simulink model "pid_bdc_z_sim"  (R2025b)
settings: Solver=ode45  StartTime=0.0  StopTime=0.5  MaxStep=0.001  RelTol=1e-3
values from neighbouring files (symbols this model uses):
  A = [-Ra/La, -Kb/La, 0 ; Kb/Je, -Be/Je, 0 ; 0, 1, 0]    [pid_bdc_z.m]
  B = [1/La ; 0 ; 0]    [pid_bdc_z.m]
  C = [0, 0, 1]    [pid_bdc_z.m]
  D = 0    [pid_bdc_z.m]
  Ts = 0.001    [pid_bdc_z.m]
libraries: cstblocks x1
settings Model: Creator=maxvega  LastModifiedBy=maxvega

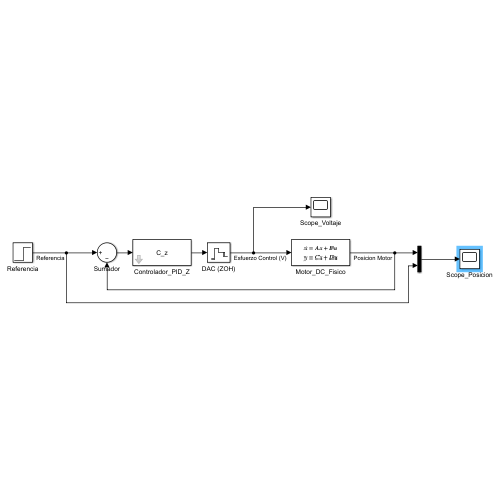
[thumbnail: Simulink's stored preview of the top-level diagram]
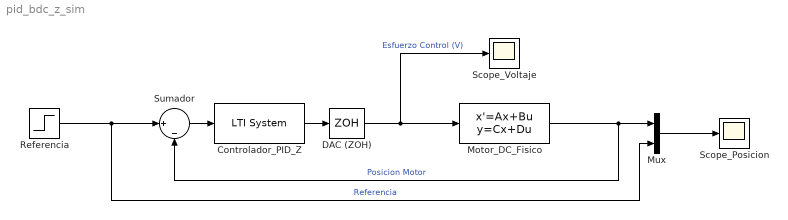
== system pid_bdc_z_sim ==
  Controlador_PID_Z : cstblocks/LTI System  sys=C_z  IC=[]  PadeOrder=0
  DAC (ZOH) : ZeroOrderHold  SampleTime=Ts
  Motor_DC_Fisico : StateSpace  A=A  B=B  C=C  D=D  InitialCondition=0
  Mux : Mux  Inputs=2
  Referencia : Step  Time=0  SampleTime=0
  Scope_Posicion : Scope
      settings: ActiveDisplayYMinimum=-0.21468036360567189  ActiveDisplayYMaximum=1.9321232724510475
  Scope_Voltaje : Scope
      settings: ActiveDisplayYMinimum=-210247.66124777796  ActiveDisplayYMaximum=248509.77533768272
  Sumador : Sum  Inputs=||+|-
  wires:
  Sumador/1 -> Controlador_PID_Z/1
  Controlador_PID_Z/1 -> DAC (ZOH)/1
  DAC (ZOH)/1 -> Motor_DC_Fisico/1, Scope_Voltaje/1  "Esfuerzo Control (V)"
  Motor_DC_Fisico/1 -> Mux/1, Sumador/2  "Posicion Motor"
  Mux/1 -> Scope_Posicion/1
  Referencia/1 -> Mux/2, Sumador/1  "Referencia"
